simulink model "sampleModel260"  (R2021b)
settings: Solver=VariableStepAuto  StartTime=0.0  StopTime=10.0  RelTol=1e-3
undefined symbols (not defined in the file or in its folder): Newton, Raphson
libraries: simulink x10, slpidlib x1
settings Model: Creator=user  LastModifiedBy=user

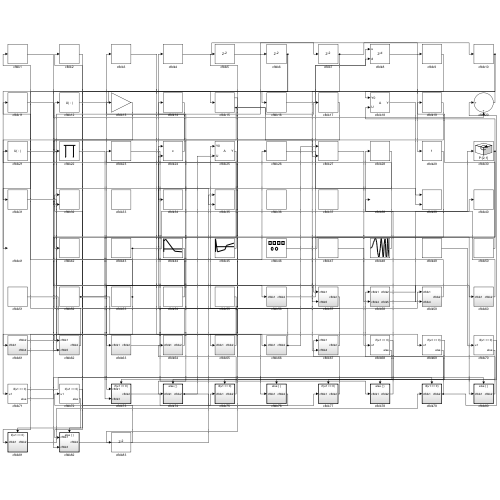
[thumbnail: Simulink's stored preview of the top-level diagram]
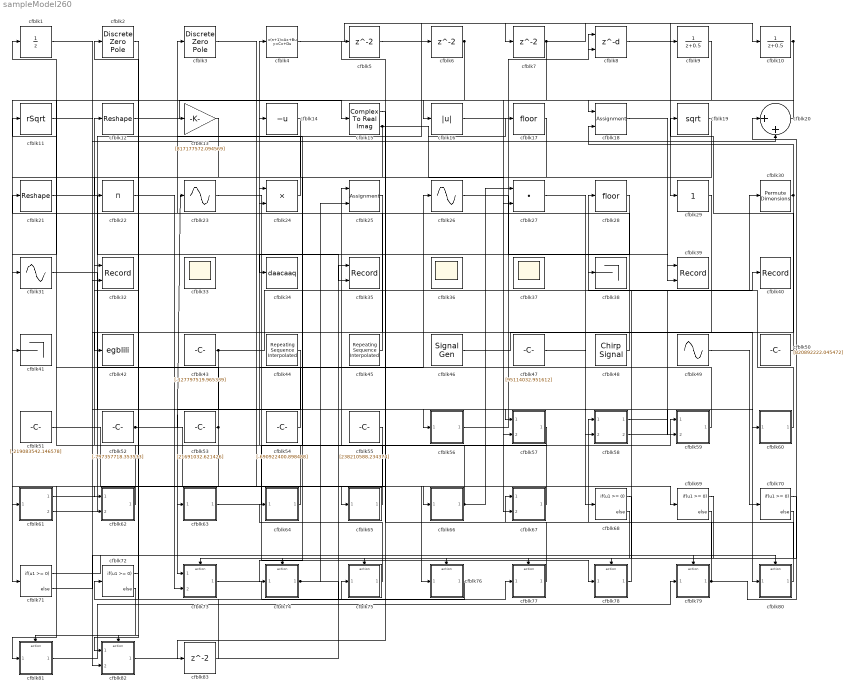
== system sampleModel260 ==
  cfblk1 : UnitDelay  HasFrameUpgradeWarning=on
  cfblk10 : DiscreteTransferFcn  SampleTime=1
  cfblk11 : Sqrt  Operator=rSqrt  AlgorithmType=Newton-Raphson  SaturateOnIntegerOverflow=on
  cfblk12 : Reshape
  cfblk13 : Gain  Gain=[817177572.094569]
  cfblk14 : UnaryMinus
  cfblk15 : ComplexToRealImag
  cfblk16 : Abs
  cfblk17 : Rounding
  cfblk18 : Assignment  DiagnosticForDimensions=Warning  IndexOptions=Index vector (dialog)  Indices=1  OutputSizes=1
  cfblk19 : Sqrt  SaturateOnIntegerOverflow=on
  cfblk2 : DiscreteZeroPole  Poles=[0 0.5]  Gain=1
  cfblk20 : Sum  Inputs=|++
  cfblk21 : Reshape
  cfblk22 : Product  Inputs=*
  cfblk23 : Sin  TimeSource=Use external signal  SampleTime=0
  cfblk24 : Product  Inputs=**
  cfblk25 : Assignment  DiagnosticForDimensions=Warning  IndexOptions=Index vector (dialog)  Indices=1  OutputSizes=1
  cfblk26 : Sin  TimeSource=Use external signal  SampleTime=0
  cfblk27 : DotProduct  InputSameDT=on  OutDataTypeStr=Inherit: Inherit via internal rule
  cfblk28 : Rounding
  cfblk29 : simulink/Math Operations/Slider Gain  gain=1  low=0  high=2
  cfblk3 : DiscreteZeroPole  Poles=[0 0.5]  Gain=1
  cfblk30 : PermuteDimensions
  cfblk31 : Sin  TimeSource=Use external signal  SampleTime=0
  cfblk32 : Record  FileSettingsInternal="{\"entries\":[{\"content\":{\"excelSettings\":{\"content\":{},\"type\":\"Streamout.ExcelSettings\"}},\"type\":\"Streamout.FileSettingStorage\",\"uuid\":\"bd282573-fbed-4e3c-a31e-0f74480bdff8\"}],\"packageUris\":[\"http://schema.mathworks.com/mf0/streamout_blocks/R2020a\"],\"version\":\"1.0\"}"  Layout=[1 1]  SignalsInternal="{\"entries\":[{\"content\":{\"signals\":[{\"content\":{\"blockPath\":[\"sampleModel260/cfblk32\"],\"channel\":[],\"dimensions\":[1],\"domain\":\"sampleModel260/cfblk32\",\"lineColor\":\"#a2142f\",\"plots\":[1],\"port\":1,\"sid\":[\"\"],\"signalID\":10815,\"signalName\":\"cfblk66\"},\"type\":\"RecordBlkView.Signal\",\"uuid\":\"2e195359-3f8a-491d-84b5-82d640c07245\"},{\"content\":{\"blockPath\":[\"sampleModel260/cfblk32\"],\"channel\":[],\"dimensions\":[1],\"domain\":\"sampleModel260/cfblk32\",\"lineColor\":\"#139fff\",\"plots\":[1],\"port\":2,\"sid\":[\"\"],\"signalID\":10819,\"signalName\":\"cfblk15:2\"},\"type\":\"RecordBlkView.Signal\",\"uuid\":\"9c70b5ea-93ee-426f-ab14-13be2462806e\"}]},\"type\":\"RecordBlkView.InputSignals\",\"uuid\":\"90f20dde-7a63-4d7e-b59c-35e4b5493080\"}],\"packageUris\":[\"http://schema.mathworks.com/mf0/streamout_blocks/R2020a\"],\"version\":\"1.0\"}"  VisualizationBindings="{\"xyplotplugin\":{\"info\":[{\"series\":[{\"bindingParametersList\":[{\"parameter\":\"X-Axis\",\"signalID\":10815,\"signalName\":\"cfblk66\"},{\"parameter\":\"Y-Axis\",\"signalID\":10819,\"signalName\":\"cfblk15:2\"}],\"seriesID\":64850}],\"subplotID\":1}]}}"  CompatibilityTag=XY
  cfblk33 : Scope
      settings: Floating=on
  cfblk34 : ToWorkspace  VariableName=daacaaq  SaveFormat=Timeseries  SampleTime=-1
  cfblk35 : Record  FileSettingsInternal="{\"entries\":[{\"content\":{\"excelSettings\":{\"content\":{},\"type\":\"Streamout.ExcelSettings\"}},\"type\":\"Streamout.FileSettingStorage\",\"uuid\":\"62094183-dbe6-4528-9498-f446f32e2bde\"}],\"packageUris\":[\"http://schema.mathworks.com/mf0/streamout_blocks/R2020a\"],\"version\":\"1.0\"}"  Layout=[1 1]  SignalsInternal="{\"entries\":[{\"content\":{\"signals\":[{\"content\":{\"blockPath\":[\"sampleModel260/cfblk35\"],\"channel\":[],\"dimensions\":[1],\"domain\":\"sampleModel260/cfblk35\",\"lineColor\":\"#a2142f\",\"plots\":[1],\"port\":1,\"sid\":[\"\"],\"signalID\":10823,\"signalName\":\"cfblk82\"},\"type\":\"RecordBlkView.Signal\",\"uuid\":\"83f55b33-c295-4031-a869-966a49bba997\"},{\"content\":{\"blockPath\":[\"sampleModel260/cfblk35\"],\"channel\":[],\"dimensions\":[1],\"domain\":\"sampleModel260/cfblk35\",\"lineColor\":\"#139fff\",\"plots\":[1],\"port\":2,\"sid\":[\"\"],\"signalID\":10827,\"signalName\":\"cfblk21\"},\"type\":\"RecordBlkView.Signal\",\"uuid\":\"9fd23f1d-01de-442e-9fdc-c009bea8f072\"}]},\"type\":\"RecordBlkView.InputSignals\",\"uuid\":\"55d6284d-6619-4c6a-aadc-de5ef6d1078c\"}],\"packageUris\":[\"http://schema.mathworks.com/mf0/streamout_blocks/R2020a\"],\"version\":\"1.0\"}"  VisualizationBindings="{\"xyplotplugin\":{\"info\":[{\"series\":[{\"bindingParametersList\":[{\"parameter\":\"X-Axis\",\"signalID\":10823,\"signalName\":\"cfblk82\"},{\"parameter\":\"Y-Axis\",\"signalID\":10827,\"signalName\":\"cfblk21\"}],\"seriesID\":13907}],\"subplotID\":1}]}}"  CompatibilityTag=XY
  cfblk36 : Scope
      settings: Floating=on
  cfblk37 : Scope
      settings: Floating=on
  cfblk38 : Terminator
  cfblk39 : Record  FileSettingsInternal="{\"entries\":[{\"content\":{\"excelSettings\":{\"content\":{},\"type\":\"Streamout.ExcelSettings\"}},\"type\":\"Streamout.FileSettingStorage\",\"uuid\":\"6d992ff3-f237-4add-b4ea-69458d49418b\"}],\"packageUris\":[\"http://schema.mathworks.com/mf0/streamout_blocks/R2020a\"],\"version\":\"1.0\"}"  Layout=[1 1]  SignalsInternal="{\"entries\":[{\"content\":{\"signals\":[{\"content\":{\"blockPath\":[\"sampleModel260/cfblk39\"],\"channel\":[],\"dimensions\":[1],\"domain\":\"sampleModel260/cfblk39\",\"lineColor\":\"#a2142f\",\"plots\":[1],\"port\":1,\"sid\":[\"\"],\"signalID\":10831,\"signalName\":\"cfblk18\"},\"type\":\"RecordBlkView.Signal\",\"uuid\":\"1a0154d0-4a65-49eb-9d4e-8549016bd023\"},{\"content\":{\"blockPath\":[\"sampleModel260/cfblk39\"],\"channel\":[],\"dimensions\":[1],\"domain\":\"sampleModel260/cfblk39\",\"lineColor\":\"#139fff\",\"plots\":[1],\"port\":2,\"sid\":[\"\"],\"signalID\":10835,\"signalName\":\"cfblk26\"},\"type\":\"RecordBlkView.Signal\",\"uuid\":\"6f94e85c-12b0-4007-93a1-2b4edfb23bb8\"}]},\"type\":\"RecordBlkView.InputSignals\",\"uuid\":\"52fa4c41-2d01-4cea-907a-678569b15f2f\"}],\"packageUris\":[\"http://schema.mathworks.com/mf0/streamout_blocks/R2020a\"],\"version\":\"1.0\"}"  VisualizationBindings="{\"xyplotplugin\":{\"info\":[{\"series\":[{\"bindingParametersList\":[{\"parameter\":\"X-Axis\",\"signalID\":10831,\"signalName\":\"cfblk18\"},{\"parameter\":\"Y-Axis\",\"signalID\":10835,\"signalName\":\"cfblk26\"}],\"seriesID\":38885}],\"subplotID\":1}]}}"  CompatibilityTag=XY
  cfblk4 : DiscreteStateSpace
  cfblk40 : Record  FileSettingsInternal="{\"entries\":[{\"content\":{\"excelSettings\":{\"content\":{},\"type\":\"Streamout.ExcelSettings\"}},\"type\":\"Streamout.FileSettingStorage\",\"uuid\":\"f35e9f53-43e7-42be-8722-fdc6e73d666a\"}],\"packageUris\":[\"http://schema.mathworks.com/mf0/streamout_blocks/R2020a\"],\"version\":\"1.0\"}"  SignalsInternal="{\"entries\":[{\"content\":{\"signals\":[{\"content\":{\"blockPath\":[\"sampleModel260/cfblk40\"],\"channel\":[],\"dimensions\":[1],\"domain\":\"sampleModel260/cfblk40\",\"lineColor\":\"#7e2f8e\",\"plots\":[1],\"port\":1,\"sid\":[\"\"],\"signalID\":10839,\"signalName\":\"cfblk58:2\"},\"type\":\"RecordBlkView.Signal\",\"uuid\":\"411b6a2f-e48e-41bc-b6cc-fb019a5a836d\"}]},\"type\":\"RecordBlkView.InputSignals\",\"uuid\":\"34515a93-7eeb-4289-942f-1bca739efc4e\"}],\"packageUris\":[\"http://schema.mathworks.com/mf0/streamout_blocks/R2020a\"],\"version\":\"1.0\"}"  VisualizationBindings="{\"sparklinesplugin\":{\"info\":[{\"bindingParametersList\":[],\"subplotID\":1}]}}"
  cfblk41 : Terminator
  cfblk42 : ToWorkspace  VariableName=egblili  SaveFormat=Timeseries  SampleTime=-1
  cfblk43 : Constant  Value=[-127797519.965339]  SampleTime=1
  cfblk44 : simulink/Sources/Repeating Sequence Interpolated  OutValues=[734542638.936509, 881551291.575524, -50590323.370308, -209229695.695795, -264688932.067042]  TimeValues=[0 0.1 0.5 0.6 1].'  LookUpMeth=Interpolation-Use End Values  tsamp=0.01  OutMin=[]  OutMax=[]  OutDataTypeStr=double  OutputDataTypeScalingMode=double  OutDataType=fixdt(0,8)  OutScaling=2^-10
  cfblk45 : simulink/Sources/Repeating Sequence Interpolated  OutValues=[975509514.452281, -690730421.354289, -411790161.170063, 161479914.581860, 466139488.744279]  TimeValues=[0 0.1 0.5 0.6 1].'  LookUpMeth=Use Input Nearest  tsamp=0.01  OutMin=[]  OutMax=[]  OutDataTypeStr=double  OutputDataTypeScalingMode=double  OutDataType=fixdt(0,8)  OutScaling=2^-10
  cfblk46 : SignalGenerator  WaveForm=square  Amplitude=[-171811111.823902]  Units=rad/sec
  cfblk47 : Constant  Value=[95114032.951612]  SampleTime=1
  cfblk48 : simulink/Sources/Chirp Signal  f1=[363968680.233004]  T=[-838285351.635962]  f2=[-356401391.651928]
  cfblk49 : Sin  Amplitude=[373258375.162552]  Bias=[-522837099.867518]  SampleTime=0
  cfblk{5..7,83} (4 alike) : Delay  SampleTime=1
  cfblk50 : Constant  Value=[820892222.045472]  SampleTime=1
  cfblk51 : Constant  Value=[-219083542.146578]  SampleTime=1
  cfblk52 : Constant  Value=[-797357718.353533]  SampleTime=1
  cfblk53 : Constant  Value=[21691032.621426]  SampleTime=1
  cfblk54 : Constant  Value=[-690922400.898488]  SampleTime=1
  cfblk55 : Constant  Value=[238210588.234374]  SampleTime=1
  cfblk56 : Subsystem
  cfblk57 : Subsystem
  cfblk58 : Subsystem
  cfblk59 : Subsystem
  cfblk60 : Subsystem
  cfblk61 : Subsystem
  cfblk62 : Subsystem
  cfblk63 : Subsystem
  cfblk64 : Subsystem
  cfblk65 : Subsystem
  cfblk66 : Subsystem
  cfblk67 : Subsystem
  cfblk{68..72} (5 alike) : If  IfExpression=u1 >= 0  SampleTime=1
  cfblk73 : Subsystem  TreatAsAtomicUnit=on
  cfblk74 : Subsystem  TreatAsAtomicUnit=on
  cfblk75 : Subsystem  TreatAsAtomicUnit=on
  cfblk76 : Subsystem  TreatAsAtomicUnit=on
  cfblk77 : Subsystem  TreatAsAtomicUnit=on
  cfblk78 : Subsystem  TreatAsAtomicUnit=on
  cfblk79 : Subsystem  TreatAsAtomicUnit=on
  cfblk8 : Delay  DelayLengthSource=Input port  SampleTime=1
      settings: InputPortMap=u0,p1
  cfblk80 : Subsystem  TreatAsAtomicUnit=on
  cfblk81 : Subsystem  TreatAsAtomicUnit=on
  cfblk82 : Subsystem  TreatAsAtomicUnit=on
  cfblk9 : DiscreteTransferFcn  SampleTime=1
  wires:
  cfblk4/1 -> cfblk10/1
  cfblk59/1(cfblk2) -> cfblk4/1
  cfblk73/1(cfblk2) -> cfblk75/1(cfblk1)
  cfblk54/1 -> cfblk24/1
  cfblk57/1(cfblk2) -> cfblk12/1
  cfblk20/1 -> cfblk16/1
  cfblk31/1 -> cfblk56/1(cfblk1)
  cfblk61/1(cfblk2) -> cfblk6/1
  cfblk46/1 -> cfblk80/1(cfblk1)
  cfblk79/1(cfblk2) -> cfblk20/1, cfblk5/1
  cfblk11/1 -> cfblk20/2
  cfblk80/1(cfblk2) -> cfblk58/1(cfblk1)
  cfblk8/1 -> cfblk29/1
  cfblk55/1 -> cfblk71/1
  cfblk65/1(cfblk2) -> cfblk25/1
  cfblk18/1 -> cfblk39/1
  cfblk77/1(cfblk2) -> cfblk67/1(cfblk1)
  cfblk24/1 -> cfblk3/1
  cfblk10/1 -> cfblk61/1(cfblk1), cfblk18/1
  cfblk16/1 -> cfblk8/1
  cfblk19/1 -> cfblk65/1(cfblk1)
  cfblk81/1(cfblk2) -> cfblk79/1(cfblk1)
  cfblk12/1 -> cfblk15/1
  cfblk56/1(cfblk2) -> cfblk8/2
  cfblk53/1 -> cfblk81/1(cfblk1), cfblk1/1
  cfblk23/1 -> cfblk78/1(cfblk1)
  cfblk14/1 -> cfblk41/1
  cfblk44/1 -> cfblk73/1(cfblk1)
  cfblk45/1 -> cfblk13/1
  cfblk7/1 -> cfblk9/1, cfblk27/2
  cfblk52/1 -> cfblk23/1, cfblk69/1
  cfblk62/1(cfblk2) -> cfblk21/1
  cfblk25/1 -> cfblk42/1
  cfblk63/1(cfblk2) -> cfblk59/1(cfblk1)
  cfblk3/1 -> cfblk66/1(cfblk1)
  cfblk58/1(cfblk2) -> cfblk60/1(cfblk1)
  cfblk75/1(cfblk2) -> cfblk64/1(cfblk1)
  cfblk47/1 -> cfblk68/1
  cfblk82/1(cfblk2) -> cfblk35/1
  cfblk61/2(cfblk4) -> cfblk26/1
  cfblk60/1(cfblk2) -> cfblk28/1
  cfblk76/1(cfblk2) -> cfblk72/1
  cfblk17/1 -> cfblk74/1(cfblk1)
  cfblk22/1 -> cfblk57/1(cfblk1)
  cfblk29/1 -> cfblk57/2(cfblk5)
  cfblk1/1 -> cfblk58/2(cfblk4)
  cfblk67/1(cfblk2) -> cfblk14/1
  cfblk51/1 -> cfblk76/1(cfblk1)
  cfblk78/1(cfblk2) -> cfblk38/1
  cfblk58/2(cfblk5) -> cfblk40/1
  cfblk30/1 -> cfblk73/2(cfblk3), cfblk62/2(cfblk5), cfblk18/2
  cfblk48/1 -> cfblk11/1
  cfblk27/1 -> cfblk59/2(cfblk4)
  cfblk74/1(cfblk2) -> cfblk77/1(cfblk1), cfblk25/2
  cfblk64/1(cfblk2) -> cfblk24/2
  cfblk21/1 -> cfblk35/2
  cfblk2/1 -> cfblk22/1
  cfblk43/1 -> cfblk63/1(cfblk1), cfblk30/1
  cfblk49/1 -> cfblk70/1
  cfblk50/1 -> cfblk19/1
  cfblk13/1 -> cfblk82/1(cfblk1)
  cfblk66/1(cfblk2) -> cfblk32/1, cfblk27/1
  cfblk5/1 -> cfblk7/1
  cfblk26/1 -> cfblk39/2
  cfblk15/2 -> cfblk17/1, cfblk67/2(cfblk4), cfblk32/2
  cfblk9/1 -> cfblk31/1
  cfblk28/1 -> cfblk34/1
  cfblk6/1 -> cfblk62/1(cfblk1), cfblk82/2(cfblk3)
  cfblk68/1 -> cfblk73/Action
  cfblk68/2 -> cfblk74/Action
  cfblk69/1 -> cfblk75/Action
  cfblk69/2 -> cfblk76/Action
  cfblk70/1 -> cfblk77/Action
  cfblk70/2 -> cfblk78/Action
  cfblk71/1 -> cfblk79/Action
  cfblk71/2 -> cfblk80/Action
  cfblk72/1 -> cfblk81/Action
  cfblk72/2 -> cfblk82/Action
  cfblk15/1 -> cfblk83/1
  cfblk83/1 -> cfblk2/1

== system sampleModel260/cfblk56 ==
  cfblk1 : Inport
  cfblk3 : Product  Inputs=*
  cfblk2 : Outport
  wires:
  cfblk1/1 -> cfblk3/1
  cfblk3/1 -> cfblk2/1

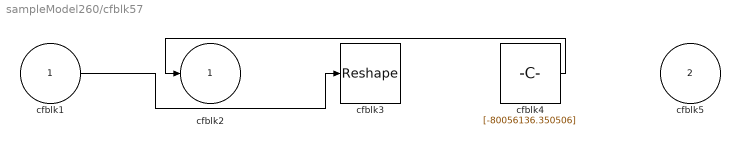
== system sampleModel260/cfblk57 ==
  cfblk1 : Inport
  cfblk5 : Inport  Port=2
  cfblk3 : Reshape
  cfblk4 : Constant  Value=[-80056136.350506]  SampleTime=1
  cfblk2 : Outport
  wires:
  cfblk4/1 -> cfblk2/1
  cfblk1/1 -> cfblk3/1

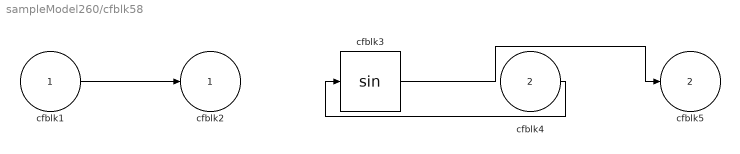
== system sampleModel260/cfblk58 ==
  cfblk1 : Inport
  cfblk4 : Inport  Port=2
  cfblk3 : Trigonometry
  cfblk2 : Outport
  cfblk5 : Outport  Port=2
  wires:
  cfblk3/1 -> cfblk5/1
  cfblk4/1 -> cfblk3/1
  cfblk1/1 -> cfblk2/1

== system sampleModel260/cfblk59 ==
  cfblk1 : Inport
  cfblk4 : Inport  Port=2
  cfblk3 : simulink/Discrete/Transfer Fcn First Order  PoleZ=0.95  ICPrevOutput=0.0  DoSatur=off
  cfblk2 : Outport
  wires:
  cfblk4/1 -> cfblk3/1
  cfblk1/1 -> cfblk2/1

== system sampleModel260/cfblk60 ==
  cfblk1 : Inport
  cfblk3 : UnaryMinus
  cfblk2 : Outport
  wires:
  cfblk3/1 -> cfblk2/1
  cfblk1/1 -> cfblk3/1

== system sampleModel260/cfblk61 ==
  cfblk1 : Inport
  cfblk3 : Constant  Value=[-179700229.476874]  SampleTime=1
  cfblk2 : Outport
  cfblk4 : Outport  Port=2
  wires:
  cfblk3/1 -> cfblk2/1
  cfblk1/1 -> cfblk4/1

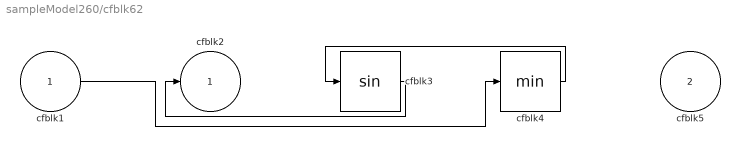
== system sampleModel260/cfblk62 ==
  cfblk1 : Inport
  cfblk5 : Inport  Port=2
  cfblk3 : Trigonometry
  cfblk4 : MinMax
  cfblk2 : Outport
  wires:
  cfblk4/1 -> cfblk3/1
  cfblk3/1 -> cfblk2/1
  cfblk1/1 -> cfblk4/1

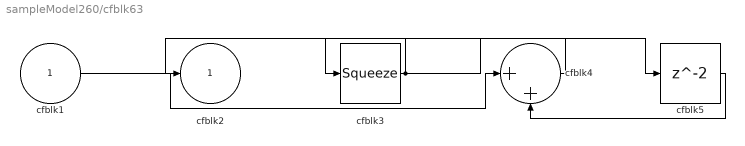
== system sampleModel260/cfblk63 ==
  cfblk1 : Inport
  cfblk3 : Squeeze
  cfblk4 : Sum  Inputs=|++
  cfblk5 : Delay  SampleTime=1
  cfblk2 : Outport
  wires:
  cfblk4/1 -> cfblk3/1
  cfblk1/1 -> cfblk4/1
  cfblk3/1 -> cfblk2/1, cfblk5/1
  cfblk5/1 -> cfblk4/2

== system sampleModel260/cfblk64 ==
  cfblk1 : Inport
  cfblk3 : DiscreteTransferFcn  SampleTime=1
  cfblk2 : Outport
  wires:
  cfblk3/1 -> cfblk2/1
  cfblk1/1 -> cfblk3/1

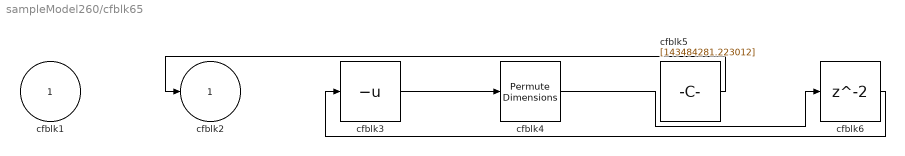
== system sampleModel260/cfblk65 ==
  cfblk1 : Inport
  cfblk3 : UnaryMinus
  cfblk4 : PermuteDimensions
  cfblk5 : Constant  Value=[143484281.223012]  SampleTime=1
  cfblk6 : Delay  SampleTime=1
  cfblk2 : Outport
  wires:
  cfblk5/1 -> cfblk2/1
  cfblk3/1 -> cfblk4/1
  cfblk4/1 -> cfblk6/1
  cfblk6/1 -> cfblk3/1

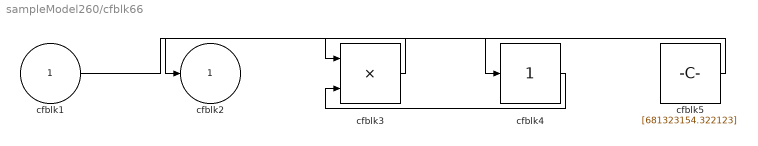
== system sampleModel260/cfblk66 ==
  cfblk1 : Inport
  cfblk3 : Product  Inputs=**
  cfblk4 : simulink/Math Operations/Slider Gain  gain=1  low=0  high=2
  cfblk5 : Constant  Value=[681323154.322123]  SampleTime=1
  cfblk2 : Outport
  wires:
  cfblk5/1 -> cfblk3/1
  cfblk4/1 -> cfblk3/2
  cfblk3/1 -> cfblk2/1
  cfblk1/1 -> cfblk4/1

== system sampleModel260/cfblk67 ==
  cfblk1 : Inport
  cfblk4 : Inport  Port=2
  cfblk3 : Sum  Inputs=+
  cfblk2 : Outport
  wires:
  cfblk1/1 -> cfblk2/1
  cfblk4/1 -> cfblk3/1

== system sampleModel260/cfblk73 ==
  cfblk1 : Inport
  cfblk3 : Inport  Port=2
  Action Port : ActionPort  ActionPortLabel=if(u1 >= 0)
  cfblk2 : Outport
  wires:
  cfblk1/1 -> cfblk2/1

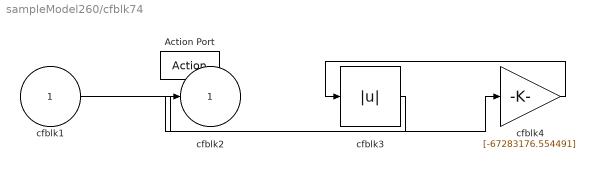
== system sampleModel260/cfblk74 ==
  cfblk1 : Inport
  Action Port : ActionPort  ActionPortLabel=else
  cfblk3 : Abs
  cfblk4 : Gain  Gain=[-67283176.554491]
  cfblk2 : Outport
  wires:
  cfblk1/1 -> cfblk4/1
  cfblk4/1 -> cfblk3/1
  cfblk3/1 -> cfblk2/1

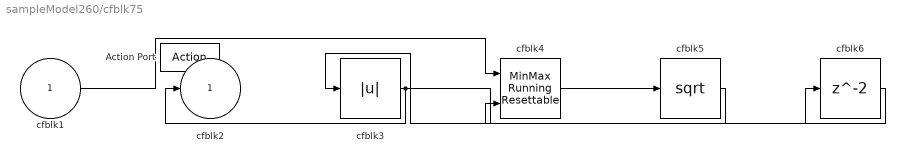
== system sampleModel260/cfblk75 ==
  cfblk1 : Inport
  Action Port : ActionPort  ActionPortLabel=if(u1 >= 0)
  cfblk3 : Abs
  cfblk4 : simulink/Math Operations/MinMax Running Resettable  Function=min  vinit=0.0
  cfblk5 : Sqrt  SaturateOnIntegerOverflow=on
  cfblk6 : Delay
  cfblk2 : Outport
  wires:
  cfblk4/1 -> cfblk5/1
  cfblk3/1 -> cfblk2/1, cfblk6/1
  cfblk1/1 -> cfblk4/1
  cfblk5/1 -> cfblk3/1
  cfblk6/1 -> cfblk4/2

== system sampleModel260/cfblk76 ==
  cfblk1 : Inport
  Action Port : ActionPort  ActionPortLabel=else
  cfblk3 : slpidlib/PID Controller  Controller=PID  Form=Parallel  TimeDomain=Discrete-time  UseExternalTs=off  SampleTime=-1  IntegratorMethod=Forward Euler  FilterMethod=Forward Euler  ControllerParametersSource=internal  P=1  I=1  D=0  UseFilter=on  N=100  TunerSelectOption=Transfer Function Based (PID Tuner App)  InitialConditionSource=internal  InitialConditionForIntegrator=0  InitialConditionForFilter=0  DifferentiatorICPrevScaledInput=0  ExternalReset=none  TrackingMode=off  Kt=1  LimitOutput=off  SatLimitsSource=internal  UpperSaturationLimit=inf  LowerSaturationLimit=-inf  LinearizeAsGain=off  AntiWindupMode=none  Kb=1  POutMin=[]  POutMax=[]  IOutMin=[]  IOutMax=[]  DOutMin=[]  DOutMax=[]  NOutMin=[]  NOutMax=[]  SumOutMin=[]  SumOutMax=[]  SaturationOutMin=[]  SaturationOutMax=[]  PParamMin=[]  PParamMax=[]  IParamMin=[]  IParamMax=[]  DParamMin=[]  DParamMax=[]  NParamMin=[]  NParamMax=[]  KbParamMin=[]  KbParamMax=[]  KtParamMin=[]  KtParamMax=[]  KbOutMin=[]  KbOutMax=[]  KtOutMin=[]  KtOutMax=[]  IntegratorOutMin=[]  IntegratorOutMax=[]  FilterOutMin=[]  FilterOutMax=[]  SumI1OutMin=[]  SumI1OutMax=[]  SumI2OutMin=[]  SumI2OutMax=[]  SumI3OutMin=[]  SumI3OutMax=[]  SumI4OutMin=[]  SumI4OutMax=[]  SumDOutMin=[]  SumDOutMax=[]  DifferentiatorOutMin=[]  DifferentiatorOutMax=[]  FilterDiffOutCoefMin=[]  FilterDiffOutCoefMax=[]  ReciprocalOutMin=[]  ReciprocalOutMax=[]  SumDenOutMin=[]  SumDenOutMax=[]  SumNumOutMin=[]  SumNumOutMax=[]  DivideOutMin=[]  DivideOutMax=[]  UdiffTsProdOutMin=[]  UdiffTsProdOutMax=[]  NTsProdOutMin=[]  NTsProdOutMax=[]  UintegralTsProdOutMin=[]  UintegralTsProdOutMax=[]  UngainTsProdOutMin=[]  UngainTsProdOutMax=[]  IntegratorContinuousStateAttributes=''  IntegratorStateMustResolveToSignalObject=off  IntegratorRTWStateStorageClass=Auto  FilterContinuousStateAttributes=''  FilterStateMustResolveToSignalObject=off  FilterRTWStateStorageClass=Auto  ParallelPVariant=InternalParameters  IdealPVariant=Disabled  IVariant=InternalParameters  DVariant=InternalParameters  IntegratorVariant=Discrete  SatVariant=Disabled  AWVariant=Passthrough  PCopyVariant=Disabled  TRVariant=Disabled  FdbkBlocksVariant=Forward  IdealPFdbkVariant=Disabled  SatFdbkVariant=Disabled  DerivativeFilterVariant=ForwardEulerFilter  NVariant=InternalParameters  NCopyVariant=Disabled  FilterICVariant=InternalICsFilter  IntegratorICVariant=InternalICs  ExternalResetVariant=Disabled  TRSumVariant=Passthrough  SumFdbkVariant=Disabled  SumVariant=Sum_PID  TsampFilterVariant=InternalTs  TsampNgainVariant=Passthrough  TsampIntegralVariant=Passthrough  ExternalSaturationOutDataTypeStr=Inherit: Same as second input
  cfblk4 : simulink/Discrete/Transfer Fcn Lead or Lag  PoleZ=0.95  ZeroZ=0.75  ICPrevOutput=0.0  ICPrevInput=0.0  DoSatur=off
      settings: SourceProductBaseCode=SL
  cfblk2 : Outport
  wires:
  cfblk4/1 -> cfblk3/1
  cfblk3/1 -> cfblk2/1
  cfblk1/1 -> cfblk4/1

== system sampleModel260/cfblk77 ==
  cfblk1 : Inport
  Action Port : ActionPort  ActionPortLabel=if(u1 >= 0)
  cfblk3 : simulink/Discrete/Transfer Fcn Lead or Lag  PoleZ=0.95  ZeroZ=0.75  ICPrevOutput=0.0  ICPrevInput=0.0  DoSatur=off
      settings: SourceProductBaseCode=SL
  cfblk2 : Outport
  wires:
  cfblk1/1 -> cfblk2/1, cfblk3/1

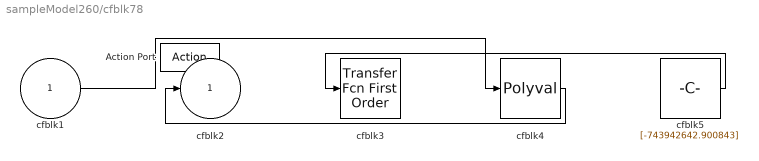
== system sampleModel260/cfblk78 ==
  cfblk1 : Inport
  Action Port : ActionPort  ActionPortLabel=else
  cfblk3 : simulink/Discrete/Transfer Fcn First Order  PoleZ=0.95  ICPrevOutput=0.0  DoSatur=off
  cfblk4 : Polyval  Coefs=[ +2.081618890e-019, -1.441693666e-014, +4.719686976e-010, -8.536869453e-006, +1.621573104e-001, -8.087801117e+001 ]
  cfblk5 : Constant  Value=[-743942642.900843]  SampleTime=1
  cfblk2 : Outport
  wires:
  cfblk4/1 -> cfblk2/1
  cfblk1/1 -> cfblk4/1
  cfblk5/1 -> cfblk3/1

== system sampleModel260/cfblk79 ==
  cfblk1 : Inport
  Action Port : ActionPort  ActionPortLabel=if(u1 >= 0)
  cfblk3 : Gain  Gain=[-1980295.320894]
  cfblk2 : Outport
  wires:
  cfblk3/1 -> cfblk2/1
  cfblk1/1 -> cfblk3/1

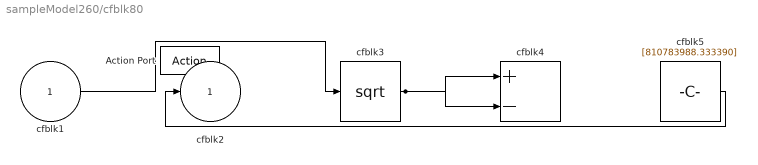
== system sampleModel260/cfblk80 ==
  cfblk1 : Inport
  Action Port : ActionPort  ActionPortLabel=else
  cfblk3 : Sqrt  SaturateOnIntegerOverflow=on
  cfblk4 : Sum  Inputs=+-
  cfblk5 : Constant  Value=[810783988.333390]  SampleTime=1
  cfblk2 : Outport
  wires:
  cfblk5/1 -> cfblk2/1
  cfblk1/1 -> cfblk3/1
  cfblk3/1 -> cfblk4/1, cfblk4/2

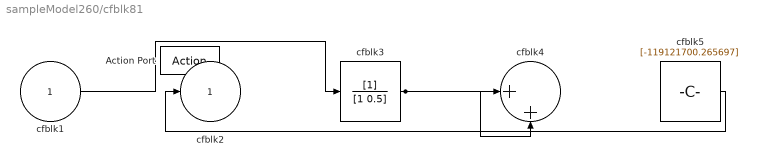
== system sampleModel260/cfblk81 ==
  cfblk1 : Inport
  Action Port : ActionPort  ActionPortLabel=if(u1 >= 0)
  cfblk3 : DiscreteFilter
  cfblk4 : Sum  Inputs=|++
  cfblk5 : Constant  Value=[-119121700.265697]  SampleTime=1
  cfblk2 : Outport
  wires:
  cfblk5/1 -> cfblk2/1
  cfblk1/1 -> cfblk3/1
  cfblk3/1 -> cfblk4/1, cfblk4/2

== system sampleModel260/cfblk82 ==
  cfblk1 : Inport
  cfblk3 : Inport  Port=2
  Action Port : ActionPort  ActionPortLabel=else
  cfblk2 : Outport
  wires:
  cfblk3/1 -> cfblk2/1
